simulink model "SIL_Autopilot_Vasarhelyi"  (R2020b)
settings: Solver=FixedStepAuto  StartTime=0  StopTime=T  FixedStep=0.01  RelTol=1e-3  EnableMultiTasking=on
model workspace (MAT data in the model file):
  SL_ROS_VariableLengthArrays_MaxSizes.CommonInfo.ArrayTruncateAction = 'EmitWarning'
  SL_ROS_VariableLengthArrays_MaxSizes.MsgTypeMap = containers.Map
  SL_ROS_VariableLengthArrays_MaxSizes.MsgTypeMap.serialization.keys = {'aircraft_communication/NetworkComm'}
  SL_ROS_VariableLengthArrays_MaxSizes.MsgTypeMap.serialization.values{1}.PropertyName = 'Comms'
  SL_ROS_VariableLengthArrays_MaxSizes.MsgTypeMap.serialization.values{1}.DataType = 'aircraft_communication/Communication'
  SL_ROS_VariableLengthArrays_MaxSizes.MsgTypeMap.serialization.values{1}.MaxLength = 5
  SL_ROS_VariableLengthArrays_MaxSizes.MsgTypeMap.serialization.uniformity = 0
  SL_ROS_VariableLengthArrays_MaxSizes.MsgTypeMap.serialization.keyType = 'char'
  SL_ROS_VariableLengthArrays_MaxSizes.MsgTypeMap.serialization.valueType = 'any'
undefined symbols (not defined in the file): Altitude_ref, DiscIntNeverNeededParam, Elevators, p_swarm, Propeller, RightAileron, RightFlap, Rudder
libraries: robotlib x20, simulink x15
(part 1 of 5)
settings Model: Creator=fcsou  LastModifiedBy=fcsou
settings OptimizationCC: EnhancedBackFolding=on  PassReuseOutputArgsAs=Individual arguments  ZeroExternalMemoryAtStartup=off  ZeroInternalMemoryAtStartup=off  MaxStackSize=64  OptimizeBlockOrder=speed  DifferentSizesBufferReuse=on  OptimizationCustomize=off  EfficientTunableParamExpr=on
settings DebuggingCC: ParameterTunabilityLossMsg=error
settings HardwareCC: ProdBitPerPointer=32  ProdBitPerSizeT=32  ProdBitPerPtrDiffT=32  ProdLargestAtomicFloat=None  ProdIntDivRoundTo=Undefined  ProdEndianess=Unspecified  ProdWordSize=32  ProdHWDeviceType=Generic->Unspecified (assume 32-bit Generic)  UseEmbeddedCoderFeatures=off
settings SFSimCC: MATLABDynamicMemAlloc=off
settings RTWCC: Description=Embedded Coder  SystemTargetFile=ert.tlc  HardwareBoard=Robot Operating System (ROS)  TLCOptions="-aInlineSetEventsForThisBaseRateFcn=TLC_FALSE -aSuppressMultiTaskScheduler=TLC_FALSE  -aRateBasedStepFcn=0"  TemplateMakefile=ert_default_tmf  Toolchain=Catkin  TargetLang=C++
settings CodeAppCC: ForceParamTrailComments=on  IgnoreCustomStorageClasses=off  OperatorAnnotations=on  SimulinkDataObjDesc=on  SFDataObjDesc=on  InsertBlockDesc=on
settings ERTTargetCC: SupportNonInlinedSFcns=on  ERTCustomFileTemplate=rostime_codertarget_file_process.tlc

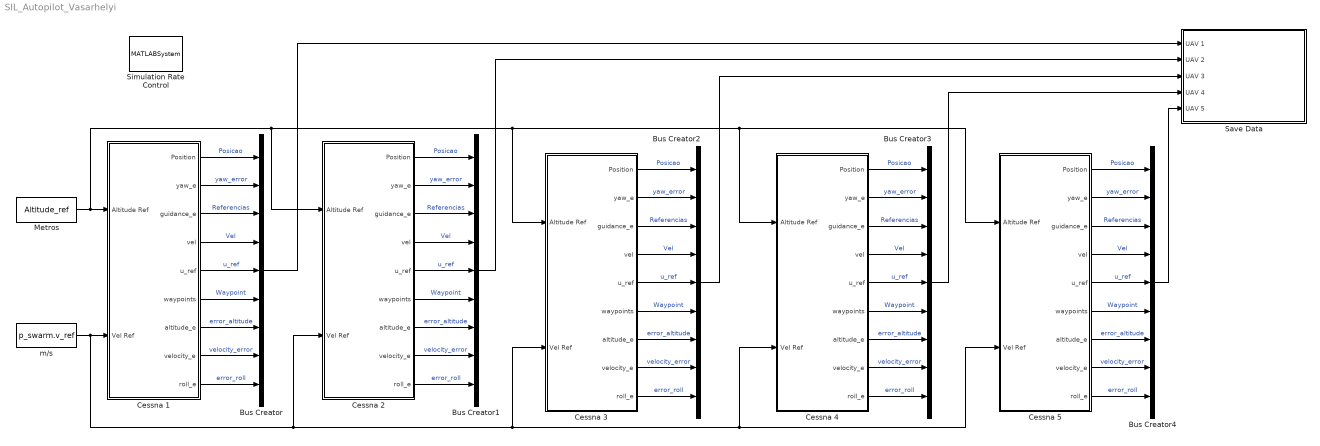
== system SIL_Autopilot_Vasarhelyi ==
  Bus Creator{,1..4} (5 alike) : BusCreator  Inputs=9
  Cessna 1 : Subsystem
  Cessna 2 : Subsystem
  Cessna 3 : Subsystem
  Cessna 4 : Subsystem
  Cessna 5 : Subsystem
  Metros : Constant  Value=Altitude_ref
  Save Data : Subsystem
  Simulation Rate Control : MATLABSystem  System=ExampleHelperSimulationRateControl  SampleTime=0.01
      mask Type: ExampleHelperSimulationRateControl
      mask Display: disp('Rate Control');
  m/s : Constant  Value=p_swarm.v_ref
  wires:
  Cessna 1/1(Position) -> Bus Creator/1  "Posicao"
  Cessna 1/2(yaw_e) -> Bus Creator/2  "yaw_error"
  Cessna 1/3(guidance_e) -> Bus Creator/3  "Referencias"
  Cessna 1/4(vel) -> Bus Creator/4  "Vel"
  Cessna 1/5(u_ref) -> Bus Creator/5  "u_ref"
  Cessna 1/6(waypoints) -> Bus Creator/6  "Waypoint"
  Cessna 1/7(altitude_e) -> Bus Creator/7  "error_altitude"
  Cessna 1/8(velocity_e) -> Bus Creator/8  "velocity_error"
  Cessna 1/9(roll_e) -> Bus Creator/9  "error_roll"
  Bus Creator/1 -> Save Data/1(UAV 1)
  Cessna 2/6(waypoints) -> Bus Creator1/6  "Waypoint"
  Cessna 2/8(velocity_e) -> Bus Creator1/8  "velocity_error"
  Cessna 2/2(yaw_e) -> Bus Creator1/2  "yaw_error"
  Cessna 2/9(roll_e) -> Bus Creator1/9  "error_roll"
  Cessna 2/5(u_ref) -> Bus Creator1/5  "u_ref"
  Cessna 2/1(Position) -> Bus Creator1/1  "Posicao"
  Cessna 2/3(guidance_e) -> Bus Creator1/3  "Referencias"
  Cessna 2/7(altitude_e) -> Bus Creator1/7  "error_altitude"
  Cessna 2/4(vel) -> Bus Creator1/4  "Vel"
  Cessna 3/6(waypoints) -> Bus Creator2/6  "Waypoint"
  Cessna 3/8(velocity_e) -> Bus Creator2/8  "velocity_error"
  Cessna 3/2(yaw_e) -> Bus Creator2/2  "yaw_error"
  Cessna 3/9(roll_e) -> Bus Creator2/9  "error_roll"
  Cessna 3/5(u_ref) -> Bus Creator2/5  "u_ref"
  Cessna 3/1(Position) -> Bus Creator2/1  "Posicao"
  Cessna 3/3(guidance_e) -> Bus Creator2/3  "Referencias"
  Cessna 3/7(altitude_e) -> Bus Creator2/7  "error_altitude"
  Cessna 3/4(vel) -> Bus Creator2/4  "Vel"
  Cessna 4/6(waypoints) -> Bus Creator3/6  "Waypoint"
  Cessna 4/8(velocity_e) -> Bus Creator3/8  "velocity_error"
  Cessna 4/2(yaw_e) -> Bus Creator3/2  "yaw_error"
  Cessna 4/9(roll_e) -> Bus Creator3/9  "error_roll"
  Cessna 4/5(u_ref) -> Bus Creator3/5  "u_ref"
  Cessna 4/1(Position) -> Bus Creator3/1  "Posicao"
  Cessna 4/3(guidance_e) -> Bus Creator3/3  "Referencias"
  Cessna 4/7(altitude_e) -> Bus Creator3/7  "error_altitude"
  Cessna 4/4(vel) -> Bus Creator3/4  "Vel"
  Metros/1 -> Cessna 5/1(Altitude Ref), Cessna 4/1(Altitude Ref), Cessna 3/1(Altitude Ref), Cessna 2/1(Altitude Ref), Cessna 1/1(Altitude Ref)
  Cessna 5/6(waypoints) -> Bus Creator4/6  "Waypoint"
  Cessna 5/8(velocity_e) -> Bus Creator4/8  "velocity_error"
  Cessna 5/2(yaw_e) -> Bus Creator4/2  "yaw_error"
  Cessna 5/9(roll_e) -> Bus Creator4/9  "error_roll"
  m/s/1 -> Cessna 3/2(Vel Ref), Cessna 4/2(Vel Ref), Cessna 5/2(Vel Ref), Cessna 2/2(Vel Ref), Cessna 1/2(Vel Ref)
  Cessna 5/5(u_ref) -> Bus Creator4/5  "u_ref"
  Cessna 5/1(Position) -> Bus Creator4/1  "Posicao"
  Cessna 5/3(guidance_e) -> Bus Creator4/3  "Referencias"
  Cessna 5/7(altitude_e) -> Bus Creator4/7  "error_altitude"
  Cessna 5/4(vel) -> Bus Creator4/4  "Vel"
  Bus Creator1/1 -> Save Data/2(UAV 2)
  Bus Creator2/1 -> Save Data/3(UAV 3)
  Bus Creator3/1 -> Save Data/4(UAV 4)
  Bus Creator4/1 -> Save Data/5(UAV 5)

== system SIL_Autopilot_Vasarhelyi/Cessna 1 ==
  Altitude Ref : Inport
  Vel Ref : Inport  Port=2
  Attitude Control : Subsystem
      settings: PortSchema="{\"entries\":[{\"content\":{\"sides\":[{\"content\":{\"connectorIds\":[\"In1\",\"In2\",\"In3\",\"In4\",\"In5\",\"In6\"]},\"type\":\"ConnectorPlacement.EquallySpacedRectSide\",\"uuid\":\"f5987fb5-26bd-460f-ada3-c62a2cc917d9\"},{\"content\":{\"connectorIds\":[\"Out1\",\"Out2\",\"Out3\",\"Out4\"],\"side\":\"RIGHT\"},\"type\":\"ConnectorPlacement.EquallySpacedRectSide\",\"uuid\":\"78b4fbb6-b2d6-45e8-a79e-ccfb1aa742fa\"},{\"content\":{\"connectorIds\":[\"Out5\",\"Out6\",\"Out7\"],\"side\":\"TOP\"},\"type\":\"ConnectorPlacement.EquallySpacedRectSide\",\"uuid\":\"043ac8db-db42-42ba-ba46-d4f45f772f93\"},{\"content\":{\"connectorIds\":[],\"side\":\"HIDDEN\"},\"type\":\"ConnectorPlacement.EquallySpacedRectSide\",\"uuid\":\"557a5d68-6739-4613-818d-4b3751c4f08a\"}]},\"type\":\"ConnectorPlacement.EquallySpacedConnector\",\"uuid\":\"675ce67f-dd1b-4b16-8fb4-2c0be5e81414\"}],\"packageUris\":[\"http://schema.mathworks.com/mf0/Connector/R2020b\"],\"version\":\"1.0\"}"
  Bus Creator : BusCreator  Inputs=3
  Bus Creator1 : BusCreator  Inputs=3
  Bus Selector1 : BusSelector  OutputSignals=X,Y
  Controle de Direção : Subsystem
  Local Flocking Algorithm : Subsystem
  ROS Communication : Subsystem
      settings: PortSchema="{\"entries\":[{\"content\":{\"sides\":[{\"content\":{\"connectorIds\":[\"In1\",\"In2\",\"In3\",\"In4\"]},\"type\":\"ConnectorPlacement.EquallySpacedRectSide\",\"uuid\":\"37ffebc2-6d57-4912-9ad0-de0bd75c512d\"},{\"content\":{\"connectorIds\":[\"Out1\",\"Out2\",\"Out3\",\"Out4\",\"Out5\",\"Out6\",\"Out7\"],\"side\":\"RIGHT\"},\"type\":\"ConnectorPlacement.EquallySpacedRectSide\",\"uuid\":\"870d0210-578f-4243-99d2-044c742eeea3\"},{\"content\":{\"connectorIds\":[\"Out8\"],\"side\":\"TOP\"},\"type\":\"ConnectorPlacement.EquallySpacedRectSide\",\"uuid\":\"d294e982-d3b3-4a84-8ae3-ca0953cabd4e\"},{\"content\":{\"connectorIds\":[],\"side\":\"HIDDEN\"},\"type\":\"ConnectorPlacement.EquallySpacedRectSide\",\"uuid\":\"f3838956-1f56-4acd-b9fa-f0f63fa39c9b\"}]},\"type\":\"ConnectorPlacement.EquallySpacedConnector\",\"uuid\":\"f2d40ee8-fbac-425c-83b3-c95127bc648e\"}],\"packageUris\":[\"http://schema.mathworks.com/mf0/Connector/R2020b\"],\"version\":\"1.0\"}"
  Position : Outport
  yaw_e : Outport  Port=2
  guidance_e : Outport  Port=3
  vel : Outport  Port=4
  u_ref : Outport  Port=5
  waypoints : Outport  Port=6
  altitude_e : Outport  Port=7
  velocity_e : Outport  Port=8
  roll_e : Outport  Port=9
  wires:
  Attitude Control/4(Throtlle) -> ROS Communication/4(Throttle)
  ROS Communication/2(Pitch) -> Bus Creator/2  "Pitch"
  Bus Selector1/2 -> Controle de Direção/3(Y)  "<Y>"
  Bus Selector1/1 -> Controle de Direção/2(X)  "<X>"
  Attitude Control/3(Aileron) -> ROS Communication/3(Aileron)
  ROS Communication/8(Xi) -> Local Flocking Algorithm/3(Xi)
  Bus Creator/1 -> Attitude Control/2(Euler Angles)
  Attitude Control/2(Rudder) -> ROS Communication/2(Rudder)
  ROS Communication/5(ECEF X) -> Bus Creator1/2  "X"
  Controle de Direção/2(Roll Ref) -> Attitude Control/3(Roll_ref)
  Attitude Control/1(Profundor) -> ROS Communication/1(Profundor)
  Bus Creator1/1 -> Position/1, Local Flocking Algorithm/1(Pos), Bus Selector1/1
  ROS Communication/6(ECEF Z) -> Attitude Control/4(Altitude), Bus Creator1/3  "Altitude"
  ROS Communication/7(Velocity) -> Attitude Control/5(Vel_in)
  Altitude Ref/1 -> Attitude Control/6(Altitude ref), Local Flocking Algorithm/2(Altitude ref)
  Local Flocking Algorithm/1(Y Ref) -> Controle de Direção/4(Y Ref)
  Local Flocking Algorithm/2(X Ref) -> Controle de Direção/5(X Ref)
  ROS Communication/3(Yaw) -> Controle de Direção/1(Yaw), Bus Creator/3  "Yaw"
  ROS Communication/4(ECEF Y) -> Bus Creator1/1  "Y"
  ROS Communication/1(Roll) -> Bus Creator/1  "Roll"
  Controle de Direção/1(yaw_error) -> yaw_e/1
  Controle de Direção/3(guidance_error) -> guidance_e/1
  Local Flocking Algorithm/3(vel) -> vel/1
  Local Flocking Algorithm/4(u_ref) -> u_ref/1
  Local Flocking Algorithm/5(Waypoints) -> waypoints/1
  Attitude Control/5(altitude_e) -> altitude_e/1
  Attitude Control/6(velocity_e) -> velocity_e/1
  Vel Ref/1 -> Attitude Control/1(Vel ref)
  Attitude Control/7(roll_e) -> roll_e/1

== system SIL_Autopilot_Vasarhelyi/Cessna 2 ==
  Altitude Ref : Inport
  Vel Ref : Inport  Port=2
  Attitude Control : Subsystem
      settings: PortSchema="{\"entries\":[{\"content\":{\"sides\":[{\"content\":{\"connectorIds\":[\"In1\",\"In2\",\"In3\",\"In4\",\"In5\",\"In6\"]},\"type\":\"ConnectorPlacement.EquallySpacedRectSide\",\"uuid\":\"f5987fb5-26bd-460f-ada3-c62a2cc917d9\"},{\"content\":{\"connectorIds\":[\"Out1\",\"Out2\",\"Out3\",\"Out4\"],\"side\":\"RIGHT\"},\"type\":\"ConnectorPlacement.EquallySpacedRectSide\",\"uuid\":\"78b4fbb6-b2d6-45e8-a79e-ccfb1aa742fa\"},{\"content\":{\"connectorIds\":[\"Out5\",\"Out6\",\"Out7\"],\"side\":\"TOP\"},\"type\":\"ConnectorPlacement.EquallySpacedRectSide\",\"uuid\":\"043ac8db-db42-42ba-ba46-d4f45f772f93\"},{\"content\":{\"connectorIds\":[],\"side\":\"HIDDEN\"},\"type\":\"ConnectorPlacement.EquallySpacedRectSide\",\"uuid\":\"557a5d68-6739-4613-818d-4b3751c4f08a\"}]},\"type\":\"ConnectorPlacement.EquallySpacedConnector\",\"uuid\":\"675ce67f-dd1b-4b16-8fb4-2c0be5e81414\"}],\"packageUris\":[\"http://schema.mathworks.com/mf0/Connector/R2020b\"],\"version\":\"1.0\"}"
  Bus Creator : BusCreator  Inputs=3
  Bus Creator1 : BusCreator  Inputs=3
  Bus Selector1 : BusSelector  OutputSignals=X,Y
  Controle de Direção : Subsystem
  Local Flocking Algorithm : Subsystem
  ROS Communication : Subsystem
      settings: PortSchema="{\"entries\":[{\"content\":{\"sides\":[{\"content\":{\"connectorIds\":[\"In1\",\"In2\",\"In3\",\"In4\"]},\"type\":\"ConnectorPlacement.EquallySpacedRectSide\",\"uuid\":\"37ffebc2-6d57-4912-9ad0-de0bd75c512d\"},{\"content\":{\"connectorIds\":[\"Out1\",\"Out2\",\"Out3\",\"Out4\",\"Out5\",\"Out6\",\"Out7\"],\"side\":\"RIGHT\"},\"type\":\"ConnectorPlacement.EquallySpacedRectSide\",\"uuid\":\"870d0210-578f-4243-99d2-044c742eeea3\"},{\"content\":{\"connectorIds\":[\"Out8\"],\"side\":\"TOP\"},\"type\":\"ConnectorPlacement.EquallySpacedRectSide\",\"uuid\":\"d294e982-d3b3-4a84-8ae3-ca0953cabd4e\"},{\"content\":{\"connectorIds\":[],\"side\":\"HIDDEN\"},\"type\":\"ConnectorPlacement.EquallySpacedRectSide\",\"uuid\":\"f3838956-1f56-4acd-b9fa-f0f63fa39c9b\"}]},\"type\":\"ConnectorPlacement.EquallySpacedConnector\",\"uuid\":\"f2d40ee8-fbac-425c-83b3-c95127bc648e\"}],\"packageUris\":[\"http://schema.mathworks.com/mf0/Connector/R2020b\"],\"version\":\"1.0\"}"
  Position : Outport
  yaw_e : Outport  Port=2
  guidance_e : Outport  Port=3
  vel : Outport  Port=4
  u_ref : Outport  Port=5
  waypoints : Outport  Port=6
  altitude_e : Outport  Port=7
  velocity_e : Outport  Port=8
  roll_e : Outport  Port=9
  wires:
  Attitude Control/4(Throtlle) -> ROS Communication/4(Throttle)
  ROS Communication/2(Pitch) -> Bus Creator/2  "Pitch"
  Bus Selector1/2 -> Controle de Direção/3(Y)  "<Y>"
  Bus Selector1/1 -> Controle de Direção/2(X)  "<X>"
  Attitude Control/3(Aileron) -> ROS Communication/3(Aileron)
  ROS Communication/8(Xi) -> Local Flocking Algorithm/3(Xi)
  Bus Creator/1 -> Attitude Control/2(Euler Angles)
  Attitude Control/2(Rudder) -> ROS Communication/2(Rudder)
  ROS Communication/5(ECEF X) -> Bus Creator1/2  "X"
  Controle de Direção/2(Roll Ref) -> Attitude Control/3(Roll_ref)
  Attitude Control/1(Profundor) -> ROS Communication/1(Profundor)
  Bus Creator1/1 -> Position/1, Local Flocking Algorithm/1(Pos), Bus Selector1/1
  ROS Communication/6(ECEF Z) -> Attitude Control/4(Altitude), Bus Creator1/3  "Altitude"
  ROS Communication/7(Velocity) -> Attitude Control/5(Vel_in)
  Altitude Ref/1 -> Attitude Control/6(Altitude ref), Local Flocking Algorithm/2(Altitude ref)
  Local Flocking Algorithm/1(Y Ref) -> Controle de Direção/4(Y Ref)
  Local Flocking Algorithm/2(X Ref) -> Controle de Direção/5(X Ref)
  ROS Communication/3(Yaw) -> Controle de Direção/1(Yaw), Bus Creator/3  "Yaw"
  ROS Communication/4(ECEF Y) -> Bus Creator1/1  "Y"
  ROS Communication/1(Roll) -> Bus Creator/1  "Roll"
  Controle de Direção/1(yaw_error) -> yaw_e/1
  Controle de Direção/3(guidance_error) -> guidance_e/1
  Local Flocking Algorithm/3(vel) -> vel/1
  Local Flocking Algorithm/4(u_ref) -> u_ref/1
  Local Flocking Algorithm/5(Waypoints) -> waypoints/1
  Attitude Control/5(altitude_e) -> altitude_e/1
  Attitude Control/6(velocity_e) -> velocity_e/1
  Vel Ref/1 -> Attitude Control/1(Vel ref)
  Attitude Control/7(roll_e) -> roll_e/1

== system SIL_Autopilot_Vasarhelyi/Cessna 3 ==
  Altitude Ref : Inport
  Vel Ref : Inport  Port=2
  Attitude Control : Subsystem
      settings: PortSchema="{\"entries\":[{\"content\":{\"sides\":[{\"content\":{\"connectorIds\":[\"In1\",\"In2\",\"In3\",\"In4\",\"In5\",\"In6\"]},\"type\":\"ConnectorPlacement.EquallySpacedRectSide\",\"uuid\":\"f5987fb5-26bd-460f-ada3-c62a2cc917d9\"},{\"content\":{\"connectorIds\":[\"Out1\",\"Out2\",\"Out3\",\"Out4\"],\"side\":\"RIGHT\"},\"type\":\"ConnectorPlacement.EquallySpacedRectSide\",\"uuid\":\"78b4fbb6-b2d6-45e8-a79e-ccfb1aa742fa\"},{\"content\":{\"connectorIds\":[\"Out5\",\"Out6\",\"Out7\"],\"side\":\"TOP\"},\"type\":\"ConnectorPlacement.EquallySpacedRectSide\",\"uuid\":\"043ac8db-db42-42ba-ba46-d4f45f772f93\"},{\"content\":{\"connectorIds\":[],\"side\":\"HIDDEN\"},\"type\":\"ConnectorPlacement.EquallySpacedRectSide\",\"uuid\":\"557a5d68-6739-4613-818d-4b3751c4f08a\"}]},\"type\":\"ConnectorPlacement.EquallySpacedConnector\",\"uuid\":\"675ce67f-dd1b-4b16-8fb4-2c0be5e81414\"}],\"packageUris\":[\"http://schema.mathworks.com/mf0/Connector/R2020b\"],\"version\":\"1.0\"}"
  Bus Creator : BusCreator  Inputs=3
  Bus Creator1 : BusCreator  Inputs=3
  Bus Selector1 : BusSelector  OutputSignals=X,Y
  Controle de Direção : Subsystem
  Local Flocking Algorithm : Subsystem
  ROS Communication : Subsystem
      settings: PortSchema="{\"entries\":[{\"content\":{\"sides\":[{\"content\":{\"connectorIds\":[\"In1\",\"In2\",\"In3\",\"In4\"]},\"type\":\"ConnectorPlacement.EquallySpacedRectSide\",\"uuid\":\"37ffebc2-6d57-4912-9ad0-de0bd75c512d\"},{\"content\":{\"connectorIds\":[\"Out1\",\"Out2\",\"Out3\",\"Out4\",\"Out5\",\"Out6\",\"Out7\"],\"side\":\"RIGHT\"},\"type\":\"ConnectorPlacement.EquallySpacedRectSide\",\"uuid\":\"870d0210-578f-4243-99d2-044c742eeea3\"},{\"content\":{\"connectorIds\":[\"Out8\"],\"side\":\"TOP\"},\"type\":\"ConnectorPlacement.EquallySpacedRectSide\",\"uuid\":\"d294e982-d3b3-4a84-8ae3-ca0953cabd4e\"},{\"content\":{\"connectorIds\":[],\"side\":\"HIDDEN\"},\"type\":\"ConnectorPlacement.EquallySpacedRectSide\",\"uuid\":\"f3838956-1f56-4acd-b9fa-f0f63fa39c9b\"}]},\"type\":\"ConnectorPlacement.EquallySpacedConnector\",\"uuid\":\"f2d40ee8-fbac-425c-83b3-c95127bc648e\"}],\"packageUris\":[\"http://schema.mathworks.com/mf0/Connector/R2020b\"],\"version\":\"1.0\"}"
  Position : Outport
  yaw_e : Outport  Port=2
  guidance_e : Outport  Port=3
  vel : Outport  Port=4
  u_ref : Outport  Port=5
  waypoints : Outport  Port=6
  altitude_e : Outport  Port=7
  velocity_e : Outport  Port=8
  roll_e : Outport  Port=9
  wires:
  Attitude Control/4(Throtlle) -> ROS Communication/4(Throttle)
  ROS Communication/2(Pitch) -> Bus Creator/2  "Pitch"
  Bus Selector1/2 -> Controle de Direção/3(Y)  "<Y>"
  Bus Selector1/1 -> Controle de Direção/2(X)  "<X>"
  Attitude Control/3(Aileron) -> ROS Communication/3(Aileron)
  ROS Communication/8(Xi) -> Local Flocking Algorithm/3(Xi)
  Bus Creator/1 -> Attitude Control/2(Euler Angles)
  Attitude Control/2(Rudder) -> ROS Communication/2(Rudder)
  ROS Communication/5(ECEF X) -> Bus Creator1/2  "X"
  Controle de Direção/2(Roll Ref) -> Attitude Control/3(Roll_ref)
  Attitude Control/1(Profundor) -> ROS Communication/1(Profundor)
  Bus Creator1/1 -> Position/1, Local Flocking Algorithm/1(Pos), Bus Selector1/1
  ROS Communication/6(ECEF Z) -> Attitude Control/4(Altitude), Bus Creator1/3  "Altitude"
  ROS Communication/7(Velocity) -> Attitude Control/5(Vel_in)
  Altitude Ref/1 -> Attitude Control/6(Altitude ref), Local Flocking Algorithm/2(Altitude ref)
  Local Flocking Algorithm/1(Y Ref) -> Controle de Direção/4(Y Ref)
  Local Flocking Algorithm/2(X Ref) -> Controle de Direção/5(X Ref)
  ROS Communication/3(Yaw) -> Controle de Direção/1(Yaw), Bus Creator/3  "Yaw"
  ROS Communication/4(ECEF Y) -> Bus Creator1/1  "Y"
  ROS Communication/1(Roll) -> Bus Creator/1  "Roll"
  Controle de Direção/1(yaw_error) -> yaw_e/1
  Controle de Direção/3(guidance_error) -> guidance_e/1
  Local Flocking Algorithm/3(vel) -> vel/1
  Local Flocking Algorithm/4(u_ref) -> u_ref/1
  Local Flocking Algorithm/5(Waypoints) -> waypoints/1
  Attitude Control/5(altitude_e) -> altitude_e/1
  Attitude Control/6(velocity_e) -> velocity_e/1
  Vel Ref/1 -> Attitude Control/1(Vel ref)
  Attitude Control/7(roll_e) -> roll_e/1

== system SIL_Autopilot_Vasarhelyi/Cessna 4 ==
  Altitude Ref : Inport
  Vel Ref : Inport  Port=2
  Attitude Control : Subsystem
      settings: PortSchema="{\"entries\":[{\"content\":{\"sides\":[{\"content\":{\"connectorIds\":[\"In1\",\"In2\",\"In3\",\"In4\",\"In5\",\"In6\"]},\"type\":\"ConnectorPlacement.EquallySpacedRectSide\",\"uuid\":\"f5987fb5-26bd-460f-ada3-c62a2cc917d9\"},{\"content\":{\"connectorIds\":[\"Out1\",\"Out2\",\"Out3\",\"Out4\"],\"side\":\"RIGHT\"},\"type\":\"ConnectorPlacement.EquallySpacedRectSide\",\"uuid\":\"78b4fbb6-b2d6-45e8-a79e-ccfb1aa742fa\"},{\"content\":{\"connectorIds\":[\"Out5\",\"Out6\",\"Out7\"],\"side\":\"TOP\"},\"type\":\"ConnectorPlacement.EquallySpacedRectSide\",\"uuid\":\"043ac8db-db42-42ba-ba46-d4f45f772f93\"},{\"content\":{\"connectorIds\":[],\"side\":\"HIDDEN\"},\"type\":\"ConnectorPlacement.EquallySpacedRectSide\",\"uuid\":\"557a5d68-6739-4613-818d-4b3751c4f08a\"}]},\"type\":\"ConnectorPlacement.EquallySpacedConnector\",\"uuid\":\"675ce67f-dd1b-4b16-8fb4-2c0be5e81414\"}],\"packageUris\":[\"http://schema.mathworks.com/mf0/Connector/R2020b\"],\"version\":\"1.0\"}"
  Bus Creator : BusCreator  Inputs=3
  Bus Creator1 : BusCreator  Inputs=3
  Bus Selector1 : BusSelector  OutputSignals=X,Y
  Controle de Direção : Subsystem
  Local Flocking Algorithm : Subsystem
  ROS Communication : Subsystem
      settings: PortSchema="{\"entries\":[{\"content\":{\"sides\":[{\"content\":{\"connectorIds\":[\"In1\",\"In2\",\"In3\",\"In4\"]},\"type\":\"ConnectorPlacement.EquallySpacedRectSide\",\"uuid\":\"37ffebc2-6d57-4912-9ad0-de0bd75c512d\"},{\"content\":{\"connectorIds\":[\"Out1\",\"Out2\",\"Out3\",\"Out4\",\"Out5\",\"Out6\",\"Out7\"],\"side\":\"RIGHT\"},\"type\":\"ConnectorPlacement.EquallySpacedRectSide\",\"uuid\":\"870d0210-578f-4243-99d2-044c742eeea3\"},{\"content\":{\"connectorIds\":[\"Out8\"],\"side\":\"TOP\"},\"type\":\"ConnectorPlacement.EquallySpacedRectSide\",\"uuid\":\"d294e982-d3b3-4a84-8ae3-ca0953cabd4e\"},{\"content\":{\"connectorIds\":[],\"side\":\"HIDDEN\"},\"type\":\"ConnectorPlacement.EquallySpacedRectSide\",\"uuid\":\"f3838956-1f56-4acd-b9fa-f0f63fa39c9b\"}]},\"type\":\"ConnectorPlacement.EquallySpacedConnector\",\"uuid\":\"f2d40ee8-fbac-425c-83b3-c95127bc648e\"}],\"packageUris\":[\"http://schema.mathworks.com/mf0/Connector/R2020b\"],\"version\":\"1.0\"}"
  Position : Outport
  yaw_e : Outport  Port=2
  guidance_e : Outport  Port=3
  vel : Outport  Port=4
  u_ref : Outport  Port=5
  waypoints : Outport  Port=6
  altitude_e : Outport  Port=7
  velocity_e : Outport  Port=8
  roll_e : Outport  Port=9
  wires:
  Attitude Control/4(Throtlle) -> ROS Communication/4(Throttle)
  ROS Communication/2(Pitch) -> Bus Creator/2  "Pitch"
  Bus Selector1/2 -> Controle de Direção/3(Y)  "<Y>"
  Bus Selector1/1 -> Controle de Direção/2(X)  "<X>"
  Attitude Control/3(Aileron) -> ROS Communication/3(Aileron)
  ROS Communication/8(Xi) -> Local Flocking Algorithm/3(Xi)
  Bus Creator/1 -> Attitude Control/2(Euler Angles)
  Attitude Control/2(Rudder) -> ROS Communication/2(Rudder)
  ROS Communication/5(ECEF X) -> Bus Creator1/2  "X"
  Controle de Direção/2(Roll Ref) -> Attitude Control/3(Roll_ref)
  Attitude Control/1(Profundor) -> ROS Communication/1(Profundor)
  Bus Creator1/1 -> Position/1, Local Flocking Algorithm/1(Pos), Bus Selector1/1
  ROS Communication/6(ECEF Z) -> Attitude Control/4(Altitude), Bus Creator1/3  "Altitude"
  ROS Communication/7(Velocity) -> Attitude Control/5(Vel_in)
  Altitude Ref/1 -> Attitude Control/6(Altitude ref), Local Flocking Algorithm/2(Altitude ref)
  Local Flocking Algorithm/1(Y Ref) -> Controle de Direção/4(Y Ref)
  Local Flocking Algorithm/2(X Ref) -> Controle de Direção/5(X Ref)
  ROS Communication/3(Yaw) -> Controle de Direção/1(Yaw), Bus Creator/3  "Yaw"
  ROS Communication/4(ECEF Y) -> Bus Creator1/1  "Y"
  ROS Communication/1(Roll) -> Bus Creator/1  "Roll"
  Controle de Direção/1(yaw_error) -> yaw_e/1
  Controle de Direção/3(guidance_error) -> guidance_e/1
  Local Flocking Algorithm/3(vel) -> vel/1
  Local Flocking Algorithm/4(u_ref) -> u_ref/1
  Local Flocking Algorithm/5(Waypoints) -> waypoints/1
  Attitude Control/5(altitude_e) -> altitude_e/1
  Attitude Control/6(velocity_e) -> velocity_e/1
  Vel Ref/1 -> Attitude Control/1(Vel ref)
  Attitude Control/7(roll_e) -> roll_e/1

== system SIL_Autopilot_Vasarhelyi/Cessna 5 ==
  Altitude Ref : Inport
  Vel Ref : Inport  Port=2
  Attitude Control : Subsystem
      settings: PortSchema="{\"entries\":[{\"content\":{\"sides\":[{\"content\":{\"connectorIds\":[\"In1\",\"In2\",\"In3\",\"In4\",\"In5\",\"In6\"]},\"type\":\"ConnectorPlacement.EquallySpacedRectSide\",\"uuid\":\"f5987fb5-26bd-460f-ada3-c62a2cc917d9\"},{\"content\":{\"connectorIds\":[\"Out1\",\"Out2\",\"Out3\",\"Out4\"],\"side\":\"RIGHT\"},\"type\":\"ConnectorPlacement.EquallySpacedRectSide\",\"uuid\":\"78b4fbb6-b2d6-45e8-a79e-ccfb1aa742fa\"},{\"content\":{\"connectorIds\":[\"Out5\",\"Out6\",\"Out7\"],\"side\":\"TOP\"},\"type\":\"ConnectorPlacement.EquallySpacedRectSide\",\"uuid\":\"043ac8db-db42-42ba-ba46-d4f45f772f93\"},{\"content\":{\"connectorIds\":[],\"side\":\"HIDDEN\"},\"type\":\"ConnectorPlacement.EquallySpacedRectSide\",\"uuid\":\"557a5d68-6739-4613-818d-4b3751c4f08a\"}]},\"type\":\"ConnectorPlacement.EquallySpacedConnector\",\"uuid\":\"675ce67f-dd1b-4b16-8fb4-2c0be5e81414\"}],\"packageUris\":[\"http://schema.mathworks.com/mf0/Connector/R2020b\"],\"version\":\"1.0\"}"
  Bus Creator : BusCreator  Inputs=3
  Bus Creator1 : BusCreator  Inputs=3
  Bus Selector1 : BusSelector  OutputSignals=X,Y
  Controle de Direção : Subsystem
  Local Flocking Algorithm : Subsystem
  ROS Communication : Subsystem
      settings: PortSchema="{\"entries\":[{\"content\":{\"sides\":[{\"content\":{\"connectorIds\":[\"In1\",\"In2\",\"In3\",\"In4\"]},\"type\":\"ConnectorPlacement.EquallySpacedRectSide\",\"uuid\":\"37ffebc2-6d57-4912-9ad0-de0bd75c512d\"},{\"content\":{\"connectorIds\":[\"Out1\",\"Out2\",\"Out3\",\"Out4\",\"Out5\",\"Out6\",\"Out7\"],\"side\":\"RIGHT\"},\"type\":\"ConnectorPlacement.EquallySpacedRectSide\",\"uuid\":\"870d0210-578f-4243-99d2-044c742eeea3\"},{\"content\":{\"connectorIds\":[\"Out8\"],\"side\":\"TOP\"},\"type\":\"ConnectorPlacement.EquallySpacedRectSide\",\"uuid\":\"d294e982-d3b3-4a84-8ae3-ca0953cabd4e\"},{\"content\":{\"connectorIds\":[],\"side\":\"HIDDEN\"},\"type\":\"ConnectorPlacement.EquallySpacedRectSide\",\"uuid\":\"f3838956-1f56-4acd-b9fa-f0f63fa39c9b\"}]},\"type\":\"ConnectorPlacement.EquallySpacedConnector\",\"uuid\":\"f2d40ee8-fbac-425c-83b3-c95127bc648e\"}],\"packageUris\":[\"http://schema.mathworks.com/mf0/Connector/R2020b\"],\"version\":\"1.0\"}"
  Position : Outport
  yaw_e : Outport  Port=2
  guidance_e : Outport  Port=3
  vel : Outport  Port=4
  u_ref : Outport  Port=5
  waypoints : Outport  Port=6
  altitude_e : Outport  Port=7
  velocity_e : Outport  Port=8
  roll_e : Outport  Port=9
  wires:
  Attitude Control/4(Throtlle) -> ROS Communication/4(Throttle)
  ROS Communication/2(Pitch) -> Bus Creator/2  "Pitch"
  Bus Selector1/2 -> Controle de Direção/3(Y)  "<Y>"
  Bus Selector1/1 -> Controle de Direção/2(X)  "<X>"
  Attitude Control/3(Aileron) -> ROS Communication/3(Aileron)
  ROS Communication/8(Xi) -> Local Flocking Algorithm/3(Xi)
  Bus Creator/1 -> Attitude Control/2(Euler Angles)
  Attitude Control/2(Rudder) -> ROS Communication/2(Rudder)
  ROS Communication/5(ECEF X) -> Bus Creator1/2  "X"
  Controle de Direção/2(Roll Ref) -> Attitude Control/3(Roll_ref)
  Attitude Control/1(Profundor) -> ROS Communication/1(Profundor)
  Bus Creator1/1 -> Position/1, Local Flocking Algorithm/1(Pos), Bus Selector1/1
  ROS Communication/6(ECEF Z) -> Attitude Control/4(Altitude), Bus Creator1/3  "Altitude"
  ROS Communication/7(Velocity) -> Attitude Control/5(Vel_in)
  Altitude Ref/1 -> Attitude Control/6(Altitude ref), Local Flocking Algorithm/2(Altitude ref)
  Local Flocking Algorithm/1(Y Ref) -> Controle de Direção/4(Y Ref)
  Local Flocking Algorithm/2(X Ref) -> Controle de Direção/5(X Ref)
  ROS Communication/3(Yaw) -> Controle de Direção/1(Yaw), Bus Creator/3  "Yaw"
  ROS Communication/4(ECEF Y) -> Bus Creator1/1  "Y"
  ROS Communication/1(Roll) -> Bus Creator/1  "Roll"
  Controle de Direção/1(yaw_error) -> yaw_e/1
  Controle de Direção/3(guidance_error) -> guidance_e/1
  Local Flocking Algorithm/3(vel) -> vel/1
  Local Flocking Algorithm/4(u_ref) -> u_ref/1
  Local Flocking Algorithm/5(Waypoints) -> waypoints/1
  Attitude Control/5(altitude_e) -> altitude_e/1
  Attitude Control/6(velocity_e) -> velocity_e/1
  Vel Ref/1 -> Attitude Control/1(Vel ref)
  Attitude Control/7(roll_e) -> roll_e/1

== system SIL_Autopilot_Vasarhelyi/Save Data ==
  UAV 1 : Inport
  UAV 2 : Inport  Port=2
  UAV 3 : Inport  Port=3
  UAV 4 : Inport  Port=4
  UAV 5 : Inport  Port=5
  To Workspace1 : ToWorkspace  VariableName=UAV1  SaveFormat=Timeseries  SampleTime=-1
  To Workspace2 : ToWorkspace  VariableName=UAV2  SaveFormat=Timeseries  SampleTime=-1
  To Workspace3 : ToWorkspace  VariableName=UAV3  SaveFormat=Timeseries  SampleTime=-1
  To Workspace4 : ToWorkspace  VariableName=UAV4  SaveFormat=Timeseries  SampleTime=-1
  To Workspace5 : ToWorkspace  VariableName=UAV5  SaveFormat=Timeseries  SampleTime=-1
  wires:
  UAV 1/1 -> To Workspace1/1
  UAV 2/1 -> To Workspace2/1
  UAV 3/1 -> To Workspace3/1
  UAV 4/1 -> To Workspace4/1
  UAV 5/1 -> To Workspace5/1

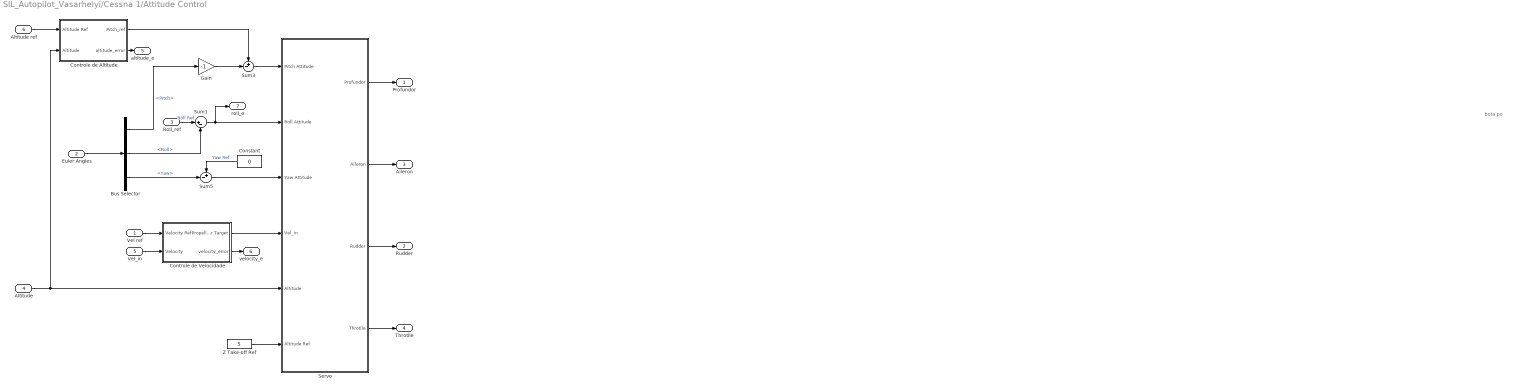
== system SIL_Autopilot_Vasarhelyi/Cessna 1/Attitude Control ==
  note: bota po
  Vel ref : Inport
  Euler Angles : Inport  Port=2
  Roll_ref : Inport  Port=3
  Altitude : Inport  Port=4
  Vel_in : Inport  Port=5
  Altitude ref : Inport  Port=6
  Bus Selector : BusSelector  OutputSignals=Pitch,Roll,Yaw
  Constant : Constant  Value=0
  Controle de Altitude : Subsystem
  Controle de Velocidade : Subsystem
  Gain : Gain  Gain=-1
  Servo : Subsystem
  Sum1 : Sum  Inputs=|+-
  Sum3 : Sum  Inputs=+-|
  Sum5 : Sum  Inputs=+-|
  Z Take-off Ref : Constant  Value=5
  Profundor : Outport
  Rudder : Outport  Port=2
  Aileron : Outport  Port=3
  Throtlle : Outport  Port=4
  altitude_e : Outport  Port=5
  velocity_e : Outport  Port=6
  roll_e : Outport  Port=7
  wires:
  Roll_ref/1 -> Sum1/1  "Roll Ref"
  Constant/1 -> Sum5/1  "Yaw Ref"
  Servo/4(Throtlle) -> Throtlle/1
  Servo/2(Aileron) -> Aileron/1
  Servo/3(Rudder) -> Rudder/1
  Servo/1(Profundor) -> Profundor/1
  Z Take-off Ref/1 -> Servo/6(Altitude Ref)
  Altitude/1 -> Controle de Altitude/2(Altitude), Servo/5(Altitude)
  Gain/1 -> Sum3/2
  Sum5/1 -> Servo/3(Yaw Attitude)
  Bus Selector/3 -> Sum5/2  "<Yaw>"
  Sum3/1 -> Servo/1(Pitch Attitude)
  Euler Angles/1 -> Bus Selector/1
  Bus Selector/1 -> Gain/1  "<Pitch>"
  Bus Selector/2 -> Sum1/2  "<Roll>"
  Controle de Velocidade/1(Propeller Target) -> Servo/4(Vel_in)
  Controle de Altitude/1(Pitch_ref) -> Sum3/1
  Vel ref/1 -> Controle de Velocidade/1(Velocity Ref)
  Altitude ref/1 -> Controle de Altitude/1(Altitude Ref)
  Sum1/1 -> roll_e/1, Servo/2(Roll Attitude)
  Vel_in/1 -> Controle de Velocidade/2(Velocity)
  Controle de Altitude/2(altitude_error) -> altitude_e/1
  Controle de Velocidade/2(velocity_error) -> velocity_e/1

== system SIL_Autopilot_Vasarhelyi/Cessna 1/Controle de Direção ==
  Yaw : Inport
  X : Inport  Port=2
  Y : Inport  Port=3
  Y Ref : Inport  Port=4
  X Ref : Inport  Port=5
  Atan2 : Trigonometry  Operator=atan2
  Discrete Derivative : simulink/Discrete/Discrete Derivative  gainval=1.0  ICPrevScaledInput=0.0  OutMin=[]  OutMax=[]  OutDataType=fixdt(1, 16)  OutScaling=2^-10  DoSatur=off
  Discrete-Time Integrator : DiscreteIntegrator  SampleTime=-1  ICPrevOutput=DiscIntNeverNeededParam  ICPrevScaledInput=DiscIntNeverNeededParam
  Kd : Gain  Gain=3.0
  Ki : Gain  Gain=0.0
  Kp : Gain  Gain=1.6616
  Mux1 : Mux  Inputs=2
  Mux2 : Mux  Inputs=2
  Mux3 : Mux  Inputs=2
  Saturation : Saturate  UpperLimit=0.226893  LowerLimit=-0.226893
  Sum2 : Sum  Inputs=|+-
  Sum3 : Sum  Inputs=|+-
  Sum4 : Sum  Inputs=|+-
  Sum5 : Sum  Inputs=+++
  neg : Gain  Gain=-1
  yaw_error : Outport
  Roll Ref : Outport  Port=2
  guidance_error : Outport  Port=3
  wires:
  Mux1/1 -> Mux3/1
  Mux2/1 -> Mux3/2
  Saturation/1 -> neg/1
  neg/1 -> Roll Ref/1
  Sum3/1 -> Atan2/1
  Y/1 -> Sum3/2, Mux2/2
  Y Ref/1 -> Sum3/1, Mux2/1
  X Ref/1 -> Sum2/1, Mux1/1
  X/1 -> Sum2/2, Mux1/2
  Sum2/1 -> Atan2/2
  Atan2/1 -> Sum4/1
  Yaw/1 -> Sum4/2
  Mux3/1 -> guidance_error/1
  Sum5/1 -> Saturation/1
  Kp/1 -> Sum5/2
  Kd/1 -> Sum5/1
  Discrete Derivative/1 -> Kd/1
  Discrete-Time Integrator/1 -> Ki/1
  Sum4/1 -> Discrete-Time Integrator/1, Kp/1, Discrete Derivative/1, yaw_error/1
  Ki/1 -> Sum5/3

== system SIL_Autopilot_Vasarhelyi/Cessna 1/Local Flocking Algorithm ==
  Pos : Inport
  Altitude ref : Inport  Port=2
  Xi : Inport  Port=3
  Bus Selector2 : BusSelector  OutputSignals=X,Y,Altitude
  Discrete Derivative : simulink/Discrete/Discrete Derivative  gainval=1.0  ICPrevScaledInput=0.0  OutMin=[]  OutMax=[]  OutDataType=fixdt(1, 16)  OutScaling=2^-10  DoSatur=off
  Gerador de Waypoints : Subsystem
  Mux : Mux  Inputs=3
  Mux1 : Mux  Inputs=3
  Vasarhelyi Algorithm : Subsystem
  Velocity Direction : MATLAB Function  TreatAsAtomicUnit=on
  Z : Display
  Y Ref : Outport
  X Ref : Outport  Port=2
  vel : Outport  Port=3
  u_ref : Outport  Port=4
  Waypoints : Outport  Port=5
  wires:
  Mux1/1 -> Waypoints/1, Velocity Direction/2(wp)
  Velocity Direction/1(u_ref) -> u_ref/1, Vasarhelyi Algorithm/3(u_ref)
  Pos/1 -> Bus Selector2/1
  Altitude ref/1 -> Mux1/3
  Gerador de Waypoints/2(Y Ref) -> Mux1/2
  Gerador de Waypoints/1(X Ref) -> Mux1/1
  Bus Selector2/1 -> Gerador de Waypoints/1(X State), Mux/1  "<X>"
  Bus Selector2/2 -> Gerador de Waypoints/2(Y State), Mux/2  "<Y>"
  Bus Selector2/3 -> Mux/3  "<Altitude>"
  Mux/1 -> Discrete Derivative/1, Vasarhelyi Algorithm/1(pos_i), Velocity Direction/1(pos)
  Discrete Derivative/1 -> vel/1
  Xi/1 -> Vasarhelyi Algorithm/2(pqj)
  Vasarhelyi Algorithm/1(X) -> X Ref/1
  Vasarhelyi Algorithm/2(Y) -> Y Ref/1
  Vasarhelyi Algorithm/3(Z) -> Z/1

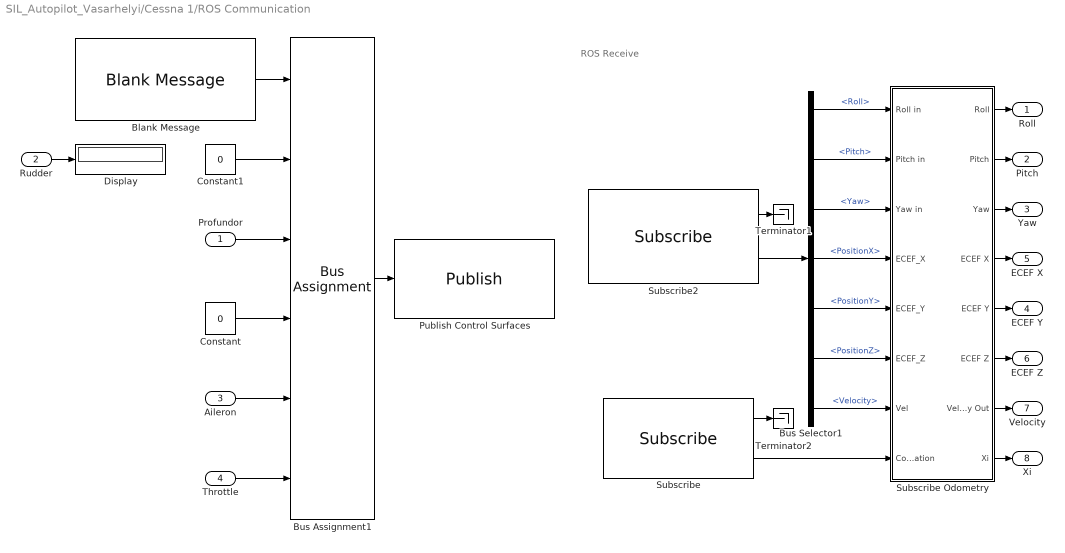
== system SIL_Autopilot_Vasarhelyi/Cessna 1/ROS Communication ==
  note: ROS Receive
  Profundor : Inport
  Rudder : Inport  Port=2
  Aileron : Inport  Port=3
  Throttle : Inport  Port=4
  Blank Message : robotlib/Blank Message  messageClass=Message  entityType=cessna_control/control_surfaces  messageType=cessna_control/control_surfaces  SampleTime=0.01  legacyBusStruct=off
  Bus Assignment1 : BusAssignment  AssignedSignals=Rudder,Elevators,RightFlap,RightAileron,Propeller
  Bus Selector1 : BusSelector  OutputSignals=Roll,Pitch,Yaw,PositionX,PositionY,PositionZ,Velocity
  Constant : Constant  Value=0
  Constant1 : Constant  Value=0
  Display : Display
  Publish Control Surfaces : robotlib/Publish  topicSource=Select from ROS network  topic=/uav1/cmd_control_surfaces  messageType=cessna_control/control_surfaces  legacyBusStruct=off  messageQueueLength=1
  Subscribe : robotlib/Subscribe  topicSource=Select from ROS network  topic=/uav1/Communication  messageType=aircraft_communication/NetworkComm  SampleTime=0.01  legacyBusStruct=off  messageQueueLength=1
  Subscribe Odometry : Subsystem  TreatAsAtomicUnit=on
  Subscribe2 : robotlib/Subscribe  topicSource=Select from ROS network  topic=/uav1/ground_truth/Odometry  messageType=aircraft_communication/Odom  SampleTime=0.01  legacyBusStruct=off  messageQueueLength=1
  Terminator1 : Terminator
  Terminator2 : Terminator
  Roll : Outport
  Pitch : Outport  Port=2
  Yaw : Outport  Port=3
  ECEF Y : Outport  Port=4
  ECEF X : Outport  Port=5
  ECEF Z : Outport  Port=6
  Velocity : Outport  Port=7
  Xi : Outport  Port=8
  wires:
  Profundor/1 -> Bus Assignment1/3
  Constant/1 -> Bus Assignment1/4
  Aileron/1 -> Bus Assignment1/5
  Subscribe Odometry/2(Pitch) -> Pitch/1
  Subscribe Odometry/4(ECEF X) -> ECEF X/1
  Subscribe Odometry/3(Yaw) -> Yaw/1
  Subscribe Odometry/1(Roll) -> Roll/1
  Subscribe Odometry/6(ECEF Z) -> ECEF Z/1
  Subscribe Odometry/7(Velocity Out) -> Velocity/1
  Rudder/1 -> Display/1
  Subscribe Odometry/8(Xi) -> Xi/1
  Throttle/1 -> Bus Assignment1/6
  Constant1/1 -> Bus Assignment1/2
  Bus Selector1/3 -> Subscribe Odometry/3(Yaw in)  "<Yaw>"
  Bus Assignment1/1 -> Publish Control Surfaces/1
  Bus Selector1/4 -> Subscribe Odometry/4(ECEF_X)  "<PositionX>"
  Bus Selector1/6 -> Subscribe Odometry/6(ECEF_Z)  "<PositionZ>"
  Blank Message/1 -> Bus Assignment1/1
  Subscribe/1 -> Terminator2/1
  Subscribe2/1 -> Terminator1/1
  Bus Selector1/2 -> Subscribe Odometry/2(Pitch in)  "<Pitch>"
  Subscribe/2 -> Subscribe Odometry/8(Communication)
  Bus Selector1/7 -> Subscribe Odometry/7(Vel)  "<Velocity>"
  Bus Selector1/1 -> Subscribe Odometry/1(Roll in)  "<Roll>"
  Bus Selector1/5 -> Subscribe Odometry/5(ECEF_Y)  "<PositionY>"
  Subscribe Odometry/5(ECEF Y) -> ECEF Y/1
  Subscribe2/2 -> Bus Selector1/1

== system SIL_Autopilot_Vasarhelyi/Cessna 2/Attitude Control ==
  note: bota po
  Vel ref : Inport
  Euler Angles : Inport  Port=2
  Roll_ref : Inport  Port=3
  Altitude : Inport  Port=4
  Vel_in : Inport  Port=5
  Altitude ref : Inport  Port=6
  Bus Selector : BusSelector  OutputSignals=Pitch,Roll,Yaw
  Constant : Constant  Value=0
  Controle de Altitude : Subsystem
  Controle de Velocidade : Subsystem
  Gain : Gain  Gain=-1
  Servo : Subsystem
  Sum1 : Sum  Inputs=|+-
  Sum3 : Sum  Inputs=+-|
  Sum5 : Sum  Inputs=+-|
  Z Take-off Ref : Constant  Value=5
  Profundor : Outport
  Rudder : Outport  Port=2
  Aileron : Outport  Port=3
  Throtlle : Outport  Port=4
  altitude_e : Outport  Port=5
  velocity_e : Outport  Port=6
  roll_e : Outport  Port=7
  wires:
  Roll_ref/1 -> Sum1/1  "Roll Ref"
  Constant/1 -> Sum5/1  "Yaw Ref"
  Servo/4(Throtlle) -> Throtlle/1
  Servo/2(Aileron) -> Aileron/1
  Servo/3(Rudder) -> Rudder/1
  Servo/1(Profundor) -> Profundor/1
  Z Take-off Ref/1 -> Servo/6(Altitude Ref)
  Altitude/1 -> Controle de Altitude/2(Altitude), Servo/5(Altitude)
  Gain/1 -> Sum3/2
  Sum5/1 -> Servo/3(Yaw Attitude)
  Bus Selector/3 -> Sum5/2  "<Yaw>"
  Sum3/1 -> Servo/1(Pitch Attitude)
  Euler Angles/1 -> Bus Selector/1
  Bus Selector/1 -> Gain/1  "<Pitch>"
  Bus Selector/2 -> Sum1/2  "<Roll>"
  Controle de Velocidade/1(Propeller Target) -> Servo/4(Vel_in)
  Controle de Altitude/1(Pitch_ref) -> Sum3/1
  Vel ref/1 -> Controle de Velocidade/1(Velocity Ref)
  Altitude ref/1 -> Controle de Altitude/1(Altitude Ref)
  Sum1/1 -> roll_e/1, Servo/2(Roll Attitude)
  Vel_in/1 -> Controle de Velocidade/2(Velocity)
  Controle de Altitude/2(altitude_error) -> altitude_e/1
  Controle de Velocidade/2(velocity_error) -> velocity_e/1

== system SIL_Autopilot_Vasarhelyi/Cessna 2/Controle de Direção ==
  Yaw : Inport
  X : Inport  Port=2
  Y : Inport  Port=3
  Y Ref : Inport  Port=4
  X Ref : Inport  Port=5
  Atan2 : Trigonometry  Operator=atan2
  Discrete Derivative : simulink/Discrete/Discrete Derivative  gainval=1.0  ICPrevScaledInput=0.0  OutMin=[]  OutMax=[]  OutDataType=fixdt(1, 16)  OutScaling=2^-10  DoSatur=off
  Discrete-Time Integrator : DiscreteIntegrator  SampleTime=-1  ICPrevOutput=DiscIntNeverNeededParam  ICPrevScaledInput=DiscIntNeverNeededParam
  Kd : Gain  Gain=3.0
  Ki : Gain  Gain=0.0
  Kp : Gain  Gain=1.6616
  Mux1 : Mux  Inputs=2
  Mux2 : Mux  Inputs=2
  Mux3 : Mux  Inputs=2
  Saturation : Saturate  UpperLimit=0.226893  LowerLimit=-0.226893
  Sum2 : Sum  Inputs=|+-
  Sum3 : Sum  Inputs=|+-
  Sum4 : Sum  Inputs=|+-
  Sum5 : Sum  Inputs=+++
  neg : Gain  Gain=-1
  yaw_error : Outport
  Roll Ref : Outport  Port=2
  guidance_error : Outport  Port=3
  wires:
  Mux1/1 -> Mux3/1
  Mux2/1 -> Mux3/2
  Saturation/1 -> neg/1
  neg/1 -> Roll Ref/1
  Sum3/1 -> Atan2/1
  Y/1 -> Sum3/2, Mux2/2
  Y Ref/1 -> Sum3/1, Mux2/1
  X Ref/1 -> Sum2/1, Mux1/1
  X/1 -> Sum2/2, Mux1/2
  Sum2/1 -> Atan2/2
  Atan2/1 -> Sum4/1
  Yaw/1 -> Sum4/2
  Mux3/1 -> guidance_error/1
  Sum5/1 -> Saturation/1
  Kp/1 -> Sum5/2
  Kd/1 -> Sum5/1
  Discrete Derivative/1 -> Kd/1
  Discrete-Time Integrator/1 -> Ki/1
  Sum4/1 -> Discrete-Time Integrator/1, Kp/1, Discrete Derivative/1, yaw_error/1
  Ki/1 -> Sum5/3

== system SIL_Autopilot_Vasarhelyi/Cessna 2/Local Flocking Algorithm ==
  Pos : Inport
  Altitude ref : Inport  Port=2
  Xi : Inport  Port=3
  Bus Selector2 : BusSelector  OutputSignals=X,Y,Altitude
  Discrete Derivative : simulink/Discrete/Discrete Derivative  gainval=1.0  ICPrevScaledInput=0.0  OutMin=[]  OutMax=[]  OutDataType=fixdt(1, 16)  OutScaling=2^-10  DoSatur=off
  Gerador de Waypoints : Subsystem
  Mux : Mux  Inputs=3
  Mux1 : Mux  Inputs=3
  Vasarhelyi Algorithm : Subsystem
  Velocity Direction : MATLAB Function  TreatAsAtomicUnit=on
  Z : Display
  Y Ref : Outport
  X Ref : Outport  Port=2
  vel : Outport  Port=3
  u_ref : Outport  Port=4
  Waypoints : Outport  Port=5
  wires:
  Mux1/1 -> Waypoints/1, Velocity Direction/2(wp)
  Velocity Direction/1(u_ref) -> u_ref/1, Vasarhelyi Algorithm/3(u_ref)
  Pos/1 -> Bus Selector2/1
  Altitude ref/1 -> Mux1/3
  Gerador de Waypoints/2(Y Ref) -> Mux1/2
  Gerador de Waypoints/1(X Ref) -> Mux1/1
  Bus Selector2/1 -> Gerador de Waypoints/1(X State), Mux/1  "<X>"
  Bus Selector2/2 -> Gerador de Waypoints/2(Y State), Mux/2  "<Y>"
  Bus Selector2/3 -> Mux/3  "<Altitude>"
  Mux/1 -> Discrete Derivative/1, Vasarhelyi Algorithm/1(pos_i), Velocity Direction/1(pos)
  Discrete Derivative/1 -> vel/1
  Xi/1 -> Vasarhelyi Algorithm/2(pqj)
  Vasarhelyi Algorithm/1(X) -> X Ref/1
  Vasarhelyi Algorithm/2(Y) -> Y Ref/1
  Vasarhelyi Algorithm/3(Z) -> Z/1

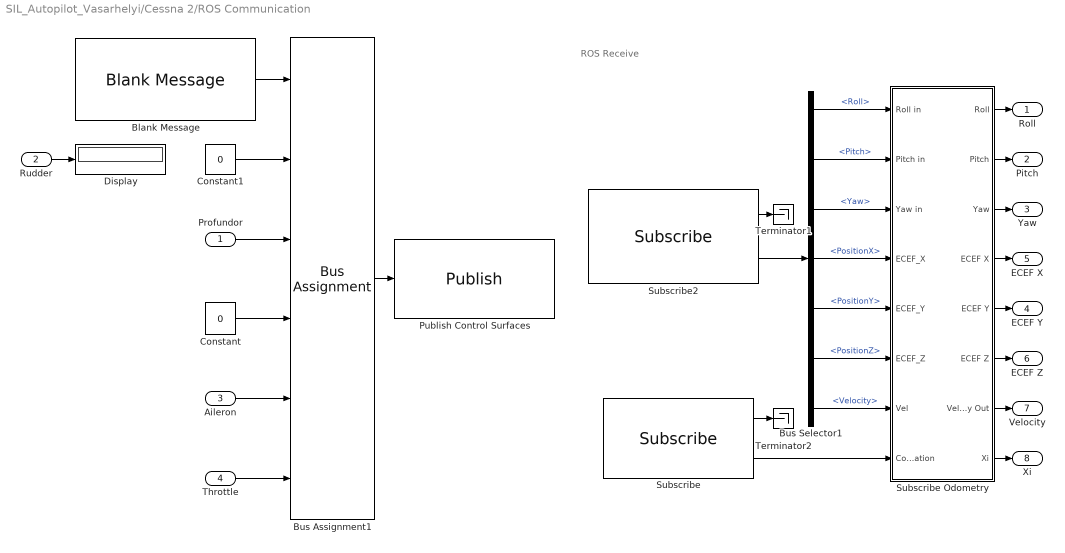
== system SIL_Autopilot_Vasarhelyi/Cessna 2/ROS Communication ==
  note: ROS Receive
  Profundor : Inport
  Rudder : Inport  Port=2
  Aileron : Inport  Port=3
  Throttle : Inport  Port=4
  Blank Message : robotlib/Blank Message  messageClass=Message  entityType=cessna_control/control_surfaces  messageType=cessna_control/control_surfaces  SampleTime=0.01  legacyBusStruct=off
  Bus Assignment1 : BusAssignment  AssignedSignals=Rudder,Elevators,RightFlap,RightAileron,Propeller
  Bus Selector1 : BusSelector  OutputSignals=Roll,Pitch,Yaw,PositionX,PositionY,PositionZ,Velocity
  Constant : Constant  Value=0
  Constant1 : Constant  Value=0
  Display : Display
  Publish Control Surfaces : robotlib/Publish  topicSource=Select from ROS network  topic=/uav2/cmd_control_surfaces  messageType=cessna_control/control_surfaces  legacyBusStruct=off  messageQueueLength=1
  Subscribe : robotlib/Subscribe  topicSource=Select from ROS network  topic=/uav2/Communication  messageType=aircraft_communication/NetworkComm  SampleTime=0.01  legacyBusStruct=off  messageQueueLength=1
  Subscribe Odometry : Subsystem  TreatAsAtomicUnit=on
  Subscribe2 : robotlib/Subscribe  topicSource=Select from ROS network  topic=/uav2/ground_truth/Odometry  messageType=aircraft_communication/Odom  SampleTime=0.01  legacyBusStruct=off  messageQueueLength=1
  Terminator1 : Terminator
  Terminator2 : Terminator
  Roll : Outport
  Pitch : Outport  Port=2
  Yaw : Outport  Port=3
  ECEF Y : Outport  Port=4
  ECEF X : Outport  Port=5
  ECEF Z : Outport  Port=6
  Velocity : Outport  Port=7
  Xi : Outport  Port=8
  wires:
  Profundor/1 -> Bus Assignment1/3
  Constant/1 -> Bus Assignment1/4
  Aileron/1 -> Bus Assignment1/5
  Subscribe Odometry/2(Pitch) -> Pitch/1
  Subscribe Odometry/4(ECEF X) -> ECEF X/1
  Subscribe Odometry/3(Yaw) -> Yaw/1
  Subscribe Odometry/1(Roll) -> Roll/1
  Subscribe Odometry/6(ECEF Z) -> ECEF Z/1
  Subscribe Odometry/7(Velocity Out) -> Velocity/1
  Rudder/1 -> Display/1
  Subscribe Odometry/8(Xi) -> Xi/1
  Throttle/1 -> Bus Assignment1/6
  Constant1/1 -> Bus Assignment1/2
  Bus Selector1/3 -> Subscribe Odometry/3(Yaw in)  "<Yaw>"
  Bus Assignment1/1 -> Publish Control Surfaces/1
  Bus Selector1/4 -> Subscribe Odometry/4(ECEF_X)  "<PositionX>"
  Bus Selector1/6 -> Subscribe Odometry/6(ECEF_Z)  "<PositionZ>"
  Blank Message/1 -> Bus Assignment1/1
  Subscribe/1 -> Terminator2/1
  Subscribe2/1 -> Terminator1/1
  Bus Selector1/2 -> Subscribe Odometry/2(Pitch in)  "<Pitch>"
  Subscribe/2 -> Subscribe Odometry/8(Communication)
  Bus Selector1/7 -> Subscribe Odometry/7(Vel)  "<Velocity>"
  Bus Selector1/1 -> Subscribe Odometry/1(Roll in)  "<Roll>"
  Bus Selector1/5 -> Subscribe Odometry/5(ECEF_Y)  "<PositionY>"
  Subscribe Odometry/5(ECEF Y) -> ECEF Y/1
  Subscribe2/2 -> Bus Selector1/1

== system SIL_Autopilot_Vasarhelyi/Cessna 3/Attitude Control ==
  note: bota po
  Vel ref : Inport
  Euler Angles : Inport  Port=2
  Roll_ref : Inport  Port=3
  Altitude : Inport  Port=4
  Vel_in : Inport  Port=5
  Altitude ref : Inport  Port=6
  Bus Selector : BusSelector  OutputSignals=Pitch,Roll,Yaw
  Constant : Constant  Value=0
  Controle de Altitude : Subsystem
  Controle de Velocidade : Subsystem
  Gain : Gain  Gain=-1
  Servo : Subsystem
  Sum1 : Sum  Inputs=|+-
  Sum3 : Sum  Inputs=+-|
  Sum5 : Sum  Inputs=+-|
  Z Take-off Ref : Constant  Value=5
  Profundor : Outport
  Rudder : Outport  Port=2
  Aileron : Outport  Port=3
  Throtlle : Outport  Port=4
  altitude_e : Outport  Port=5
  velocity_e : Outport  Port=6
  roll_e : Outport  Port=7
  wires:
  Roll_ref/1 -> Sum1/1  "Roll Ref"
  Constant/1 -> Sum5/1  "Yaw Ref"
  Servo/4(Throtlle) -> Throtlle/1
  Servo/2(Aileron) -> Aileron/1
  Servo/3(Rudder) -> Rudder/1
  Servo/1(Profundor) -> Profundor/1
  Z Take-off Ref/1 -> Servo/6(Altitude Ref)
  Altitude/1 -> Controle de Altitude/2(Altitude), Servo/5(Altitude)
  Gain/1 -> Sum3/2
  Sum5/1 -> Servo/3(Yaw Attitude)
  Bus Selector/3 -> Sum5/2  "<Yaw>"
  Sum3/1 -> Servo/1(Pitch Attitude)
  Euler Angles/1 -> Bus Selector/1
  Bus Selector/1 -> Gain/1  "<Pitch>"
  Bus Selector/2 -> Sum1/2  "<Roll>"
  Controle de Velocidade/1(Propeller Target) -> Servo/4(Vel_in)
  Controle de Altitude/1(Pitch_ref) -> Sum3/1
  Vel ref/1 -> Controle de Velocidade/1(Velocity Ref)
  Altitude ref/1 -> Controle de Altitude/1(Altitude Ref)
  Sum1/1 -> roll_e/1, Servo/2(Roll Attitude)
  Vel_in/1 -> Controle de Velocidade/2(Velocity)
  Controle de Altitude/2(altitude_error) -> altitude_e/1
  Controle de Velocidade/2(velocity_error) -> velocity_e/1

== system SIL_Autopilot_Vasarhelyi/Cessna 3/Controle de Direção ==
  Yaw : Inport
  X : Inport  Port=2
  Y : Inport  Port=3
  Y Ref : Inport  Port=4
  X Ref : Inport  Port=5
  Atan2 : Trigonometry  Operator=atan2
  Discrete Derivative : simulink/Discrete/Discrete Derivative  gainval=1.0  ICPrevScaledInput=0.0  OutMin=[]  OutMax=[]  OutDataType=fixdt(1, 16)  OutScaling=2^-10  DoSatur=off
  Discrete-Time Integrator : DiscreteIntegrator  SampleTime=-1  ICPrevOutput=DiscIntNeverNeededParam  ICPrevScaledInput=DiscIntNeverNeededParam
  Kd : Gain  Gain=3.0
  Ki : Gain  Gain=0.0
  Kp : Gain  Gain=1.6616
  Mux1 : Mux  Inputs=2
  Mux2 : Mux  Inputs=2
  Mux3 : Mux  Inputs=2
  Saturation : Saturate  UpperLimit=0.226893  LowerLimit=-0.226893
  Sum2 : Sum  Inputs=|+-
  Sum3 : Sum  Inputs=|+-
  Sum4 : Sum  Inputs=|+-
  Sum5 : Sum  Inputs=+++
  neg : Gain  Gain=-1
  yaw_error : Outport
  Roll Ref : Outport  Port=2
  guidance_error : Outport  Port=3
  wires:
  Mux1/1 -> Mux3/1
  Mux2/1 -> Mux3/2
  Saturation/1 -> neg/1
  neg/1 -> Roll Ref/1
  Sum3/1 -> Atan2/1
  Y/1 -> Sum3/2, Mux2/2
  Y Ref/1 -> Sum3/1, Mux2/1
  X Ref/1 -> Sum2/1, Mux1/1
  X/1 -> Sum2/2, Mux1/2
  Sum2/1 -> Atan2/2
  Atan2/1 -> Sum4/1
  Yaw/1 -> Sum4/2
  Mux3/1 -> guidance_error/1
  Sum5/1 -> Saturation/1
  Kp/1 -> Sum5/2
  Kd/1 -> Sum5/1
  Discrete Derivative/1 -> Kd/1
  Discrete-Time Integrator/1 -> Ki/1
  Sum4/1 -> Discrete-Time Integrator/1, Kp/1, Discrete Derivative/1, yaw_error/1
  Ki/1 -> Sum5/3

== system SIL_Autopilot_Vasarhelyi/Cessna 3/Local Flocking Algorithm ==
  Pos : Inport
  Altitude ref : Inport  Port=2
  Xi : Inport  Port=3
  Bus Selector2 : BusSelector  OutputSignals=X,Y,Altitude
  Discrete Derivative : simulink/Discrete/Discrete Derivative  gainval=1.0  ICPrevScaledInput=0.0  OutMin=[]  OutMax=[]  OutDataType=fixdt(1, 16)  OutScaling=2^-10  DoSatur=off
  Gerador de Waypoints : Subsystem
  Mux : Mux  Inputs=3
  Mux1 : Mux  Inputs=3
  Vasarhelyi Algorithm : Subsystem
  Velocity Direction : MATLAB Function  TreatAsAtomicUnit=on
  Z : Display
  Y Ref : Outport
  X Ref : Outport  Port=2
  vel : Outport  Port=3
  u_ref : Outport  Port=4
  Waypoints : Outport  Port=5
  wires:
  Mux1/1 -> Waypoints/1, Velocity Direction/2(wp)
  Velocity Direction/1(u_ref) -> u_ref/1, Vasarhelyi Algorithm/3(u_ref)
  Pos/1 -> Bus Selector2/1
  Altitude ref/1 -> Mux1/3
  Gerador de Waypoints/2(Y Ref) -> Mux1/2
  Gerador de Waypoints/1(X Ref) -> Mux1/1
  Bus Selector2/1 -> Gerador de Waypoints/1(X State), Mux/1  "<X>"
  Bus Selector2/2 -> Gerador de Waypoints/2(Y State), Mux/2  "<Y>"
  Bus Selector2/3 -> Mux/3  "<Altitude>"
  Mux/1 -> Discrete Derivative/1, Vasarhelyi Algorithm/1(pos_i), Velocity Direction/1(pos)
  Discrete Derivative/1 -> vel/1
  Xi/1 -> Vasarhelyi Algorithm/2(pqj)
  Vasarhelyi Algorithm/1(X) -> X Ref/1
  Vasarhelyi Algorithm/2(Y) -> Y Ref/1
  Vasarhelyi Algorithm/3(Z) -> Z/1

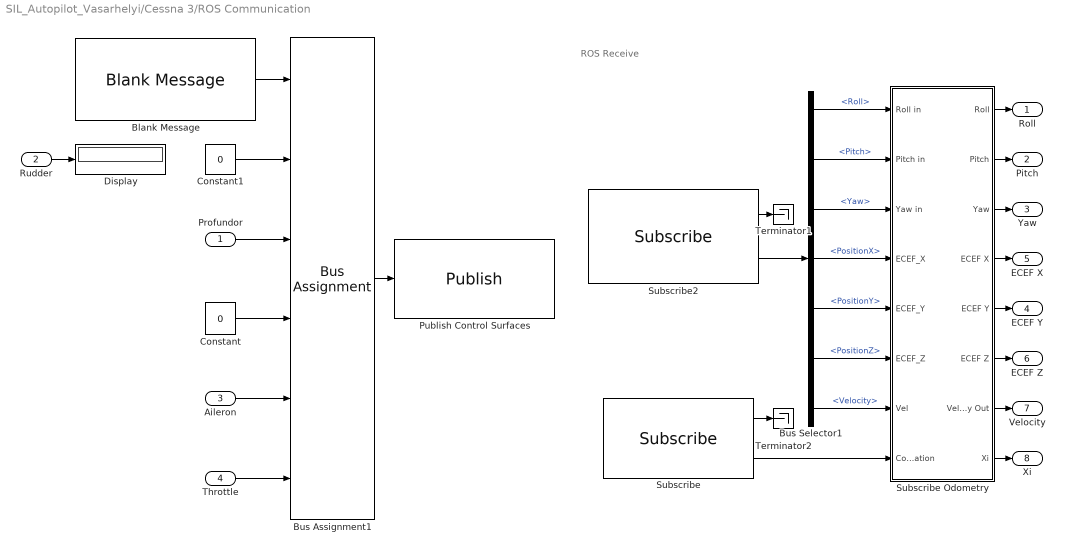
== system SIL_Autopilot_Vasarhelyi/Cessna 3/ROS Communication ==
  note: ROS Receive
  Profundor : Inport
  Rudder : Inport  Port=2
  Aileron : Inport  Port=3
  Throttle : Inport  Port=4
  Blank Message : robotlib/Blank Message  messageClass=Message  entityType=cessna_control/control_surfaces  messageType=cessna_control/control_surfaces  SampleTime=0.01  legacyBusStruct=off
  Bus Assignment1 : BusAssignment  AssignedSignals=Rudder,Elevators,RightFlap,RightAileron,Propeller
  Bus Selector1 : BusSelector  OutputSignals=Roll,Pitch,Yaw,PositionX,PositionY,PositionZ,Velocity
  Constant : Constant  Value=0
  Constant1 : Constant  Value=0
  Display : Display
  Publish Control Surfaces : robotlib/Publish  topicSource=Select from ROS network  topic=/uav3/cmd_control_surfaces  messageType=cessna_control/control_surfaces  legacyBusStruct=off  messageQueueLength=1
  Subscribe : robotlib/Subscribe  topicSource=Select from ROS network  topic=/uav3/Communication  messageType=aircraft_communication/NetworkComm  SampleTime=0.01  legacyBusStruct=off  messageQueueLength=1
  Subscribe Odometry : Subsystem  TreatAsAtomicUnit=on
  Subscribe2 : robotlib/Subscribe  topicSource=Select from ROS network  topic=/uav3/ground_truth/Odometry  messageType=aircraft_communication/Odom  SampleTime=0.01  legacyBusStruct=off  messageQueueLength=1
  Terminator1 : Terminator
  Terminator2 : Terminator
  Roll : Outport
  Pitch : Outport  Port=2
  Yaw : Outport  Port=3
  ECEF Y : Outport  Port=4
  ECEF X : Outport  Port=5
  ECEF Z : Outport  Port=6
  Velocity : Outport  Port=7
  Xi : Outport  Port=8
  wires:
  Profundor/1 -> Bus Assignment1/3
  Constant/1 -> Bus Assignment1/4
  Aileron/1 -> Bus Assignment1/5
  Subscribe Odometry/2(Pitch) -> Pitch/1
  Subscribe Odometry/4(ECEF X) -> ECEF X/1
  Subscribe Odometry/3(Yaw) -> Yaw/1
  Subscribe Odometry/1(Roll) -> Roll/1
  Subscribe Odometry/6(ECEF Z) -> ECEF Z/1
  Subscribe Odometry/7(Velocity Out) -> Velocity/1
  Rudder/1 -> Display/1
  Subscribe Odometry/8(Xi) -> Xi/1
  Throttle/1 -> Bus Assignment1/6
  Constant1/1 -> Bus Assignment1/2
  Bus Selector1/3 -> Subscribe Odometry/3(Yaw in)  "<Yaw>"
  Bus Assignment1/1 -> Publish Control Surfaces/1
  Bus Selector1/4 -> Subscribe Odometry/4(ECEF_X)  "<PositionX>"
  Bus Selector1/6 -> Subscribe Odometry/6(ECEF_Z)  "<PositionZ>"
  Blank Message/1 -> Bus Assignment1/1
  Subscribe/1 -> Terminator2/1
  Subscribe2/1 -> Terminator1/1
  Bus Selector1/2 -> Subscribe Odometry/2(Pitch in)  "<Pitch>"
  Subscribe/2 -> Subscribe Odometry/8(Communication)
  Bus Selector1/7 -> Subscribe Odometry/7(Vel)  "<Velocity>"
  Bus Selector1/1 -> Subscribe Odometry/1(Roll in)  "<Roll>"
  Bus Selector1/5 -> Subscribe Odometry/5(ECEF_Y)  "<PositionY>"
  Subscribe Odometry/5(ECEF Y) -> ECEF Y/1
  Subscribe2/2 -> Bus Selector1/1
